simulink model "CommsOutMAV"  (R2026a)
settings: Solver=VariableStepAuto
undefined symbols (not defined in the file): ts_uav
libraries: uavmavlinklib x2
settings Model: DataDictionary=QuadData.sldd  Creator=The MathWorks, Inc.  LastModifiedBy=The MathWorks, Inc.

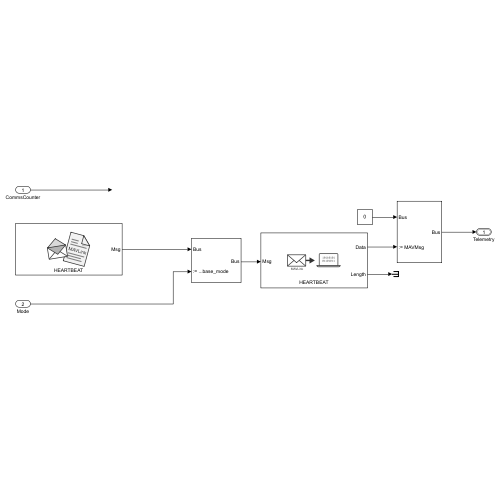
[thumbnail: Simulink's stored preview of the top-level diagram]
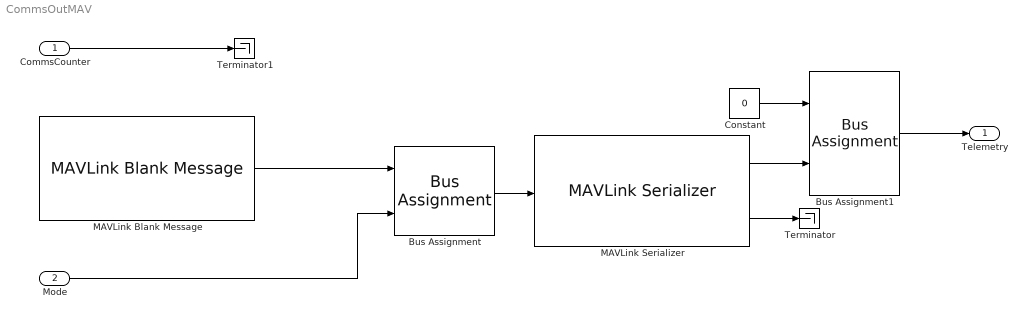
== system CommsOutMAV ==
  CommsCounter : Inport  OutDataTypeStr=uint8  PortDimensions=1
  Mode : Inport  Port=2
  Bus Assignment : BusAssignment  AssignedSignals=Payload.base_mode
  Bus Assignment1 : BusAssignment  AssignedSignals=MAVMsg
  Constant : Constant  Value=0  OutDataTypeStr=Bus: Telemetry
  MAVLink Blank Message : uavmavlinklib/MAVLink Blank Message  dialectSource=Select from standard MAVLink dialects  dialect=common.xml  dialectCustom=common.xml  version=2  messageType=HEARTBEAT  SystemID=1  ComponentID=1  SampleTime=ts_uav
  MAVLink Serializer : uavmavlinklib/MAVLink Serializer  dialectSource=Select from standard MAVLink dialects  dialect=common.xml  dialectCustom=common.xml  version=2  messageType=HEARTBEAT
  Terminator : Terminator
  Terminator1 : Terminator
  Telemetry : Outport  OutDataTypeStr=Bus: Telemetry
  wires:
  MAVLink Serializer/2 -> Terminator/1
  MAVLink Blank Message/1 -> Bus Assignment/1
  Bus Assignment/1 -> MAVLink Serializer/1
  Mode/1 -> Bus Assignment/2
  Bus Assignment1/1 -> Telemetry/1
  MAVLink Serializer/1 -> Bus Assignment1/2
  Constant/1 -> Bus Assignment1/1
  CommsCounter/1 -> Terminator1/1
